simulink model "Controllo_CG"  (R2014b)
settings: Solver=ode45  SolverMode=SingleTasking  StartTime=0.0  StopTime=10.0  RelTol=1e-3
values from neighbouring files (symbols this model uses):
  b = size(G,2)    [OffsetFree.m]    (also in main.m = [qmax -qmin hmax -hmin Fmax -Fmin]')
  delta = 1e-3    (= 0.001)    [main.m]
  F_lq = F_aug(1,1:dimA(1))    [LQI_control.m]
  Fhi = sysTotal.a    [main.m]
  G = sysTotal.b    [main.m]
  Hc = [1 0 0 0 0; 0 1 0 0 0; -F_lq Ci]    [main.m]
  k0 = horizon    [calcola_k0.m]    (also in main.m = 35)
  L = [sysTotal.d; zeros(nc-1,1)]    [main.m]
  par = [1 5 1.5 4 20 0.5 1 0.5]    [main.m]
  Riferimento = [0 0 0 0 0 0 0 0 0 0 0 0 ... (1000 elements, 1x1000)]    [ref.mat]
  T = [1 0 0; -1 0 0; 0 1 0; 0 -1 0; 0 0 1; 0 0 -1]    [main.m]
  Ts = 0.01    [main.m]
  ueq = m2*g + (k2 + k1/R^2)*heq    [main.m]
  x0 = zeros(size(Ad,1),1)    [LQI_control.m]    (also in main.m = [0 0 0 0]')
  xeq = [0 0 -g*L*m1*R/k1 0]    [main.m]
undefined symbols (not defined in the file or in its folder): Ai, Bi, Calcolo_CG, Ci, Di
settings Model: CovSFcnEnable=on  Creator=Piero  LastModifiedBy=Gianni
settings OptimizationCC: BlockReduction=off  BooleanDataType=off  UseDivisionForNetSlopeComputation=off  SimCompilerOptimization=off
settings DebuggingCC: SaveWithParameterizedLinksMsg=none  UnderspecifiedInitializationDetection=Classic  MergeDetectMultiDrivingBlocksExec=none  SignalResolutionControl=TryResolveAllWithWarning  SolverPrmCheckMsg=none  FrameProcessingCompatibilityMsg=error
settings HardwareCC: TargetUnknown=on
settings RTWCC: RTWCompilerOptimization=off

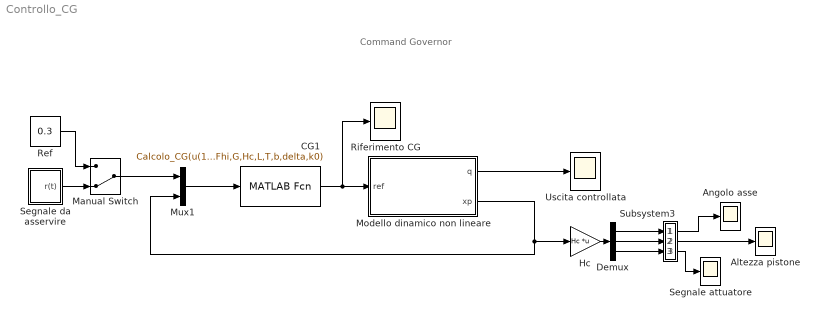
== system Controllo_CG ==
  note: Command Governor
  Altezza pistone : Scope
      settings: TimeRange=10  YMin=-1  YMax=1  SaveName=h_CG
  Angolo asse : Scope
      settings: YMin=-0.5  YMax=0.5  SaveName=q_CG
  CG1 : MATLABFcn  MATLABFcn=Calcolo_CG(u(1),u(2:6),Fhi,G,Hc,L,T,b,delta,k0)  OutputDimensions=1  SampleTime=Ts
  Demux : Demux  Outputs=3
  Hc : Gain  Gain=Hc  Multiplication=Matrix(K*u)
  Manual Switch : ManualSwitch  CurrentSetting=0
  Modello dinamico non lineare : Subsystem
  Mux1 : Mux  Inputs=2
  Ref : Constant  Value=0.3
  Riferimento CG : Scope
      settings: YMin=0.04795  YMax=0.049  SaveName=ref_CG
  Segnale attuatore : Scope
      settings: TimeRange=10  YMin=-8.353816285490428  YMax=-5.295925289307348  SaveName=u_CG
  Segnale da asservire : Subsystem
  Subsystem3 : Subsystem
      mask Display: port_label('output', 1, '')
  "Uscita controllata " : Scope
      settings: YMin=0.09  YMax=0.1325
  wires:
  Modello dinamico non lineare/2(xp) -> Mux1/2, Hc/1
  Modello dinamico non lineare/1(q) -> "Uscita controllata "/1
  Hc/1 -> Demux/1
  Manual Switch/1 -> Mux1/1
  Demux/1 -> Subsystem3/1(z)
  Demux/2 -> Subsystem3/2(h)
  Demux/3 -> Subsystem3/3(F)
  Subsystem3/1(z_vinc) -> Angolo asse/1
  Subsystem3/2(h_vinc) -> Altezza pistone/1
  Subsystem3/3(F_vinc) -> Segnale attuatore/1
  Segnale da asservire/1(r(t)) -> Manual Switch/2
  Ref/1 -> Manual Switch/1
  Mux1/1 -> CG1/1
  CG1/1 -> Riferimento CG/1, Modello dinamico non lineare/1(ref)

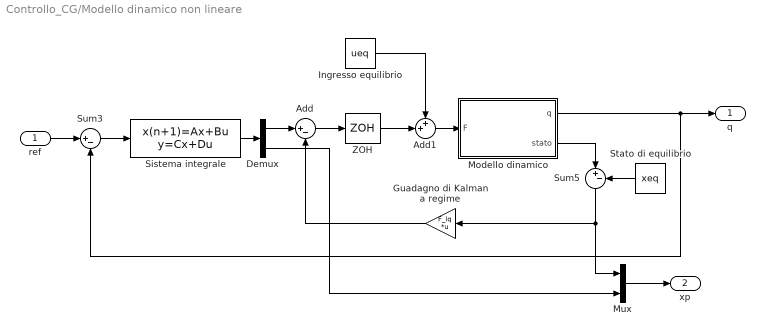
== system Controllo_CG/Modello dinamico non lineare ==
  ref : Inport
  Add : Sum  Inputs=|+-
  Add1 : Sum  Inputs=++|
  Demux : Demux  Outputs=2
  Guadagno di Kalman a regime : Gain  Gain=F_lq  Multiplication=Matrix(K*u) (u vector)
  Ingresso equilibrio : Constant  Value=ueq
  Modello dinamico : Subsystem
  Mux : Mux  Inputs=2
  Sistema integrale : DiscreteStateSpace  A=Ai  B=Bi  C=[Ci;1]  D=[Di;0]  SampleTime=Ts
  Stato di equilibrio : Constant  Value=xeq
  Sum3 : Sum  Inputs=|+-
  Sum5 : Sum  Inputs=|+-
  ZOH : ZeroOrderHold  SampleTime=Ts
  q : Outport
  xp : Outport  Port=2
  wires:
  Demux/2 -> Mux/2
  Sistema integrale/1 -> Demux/1
  Mux/1 -> xp/1
  Sum3/1 -> Sistema integrale/1
  Stato di equilibrio/1 -> Sum5/2
  ZOH/1 -> Add1/2
  Modello dinamico/1(q) -> Sum3/2, q/1
  Add/1 -> ZOH/1
  Modello dinamico/2(stato) -> Sum5/1
  ref/1 -> Sum3/1
  Add1/1 -> Modello dinamico/1("F ")
  Demux/1 -> Add/1
  Guadagno di Kalman a regime/1 -> Add/2
  Ingresso equilibrio/1 -> Add1/1
  Sum5/1 -> Mux/1, Guadagno di Kalman a regime/1

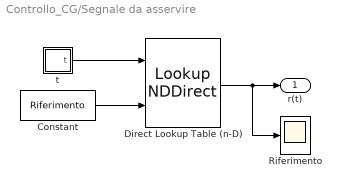
== system Controllo_CG/Segnale da asservire ==
  Constant : Constant  Value=Riferimento
  Direct Lookup Table (n-D) : LookupNDDirect  NumberOfTableDimensions=1  TableIsInput=on
  Riferimento : Scope
      settings: YMin=0.3995  YMax=0.3998  SaveName=ref
  t : Subsystem
  r(t) : Outport
  wires:
  Constant/1 -> Direct Lookup Table (n-D)/2
  t/1(t) -> Direct Lookup Table (n-D)/1
  Direct Lookup Table (n-D)/1 -> Riferimento/1, r(t)/1

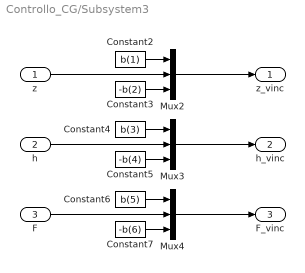
== system Controllo_CG/Subsystem3 ==
  z : Inport
  h : Inport  Port=2
  F : Inport  Port=3
  Constant2 : Constant  Value=b(1)
  Constant3 : Constant  Value=-b(2)
  Constant4 : Constant  Value=b(3)
  Constant5 : Constant  Value=-b(4)
  Constant6 : Constant  Value=b(5)
  Constant7 : Constant  Value=-b(6)
  Mux2 : Mux  Inputs=3
  Mux3 : Mux  Inputs=3
  Mux4 : Mux  Inputs=3
  z_vinc : Outport
  h_vinc : Outport  Port=2
  F_vinc : Outport  Port=3
  wires:
  h/1 -> Mux3/2
  Mux2/1 -> z_vinc/1
  F/1 -> Mux4/2
  Constant3/1 -> Mux2/3
  Constant2/1 -> Mux2/1
  z/1 -> Mux2/2
  Constant4/1 -> Mux3/1
  Constant5/1 -> Mux3/3
  Constant6/1 -> Mux4/1
  Constant7/1 -> Mux4/3
  Mux3/1 -> h_vinc/1
  Mux4/1 -> F_vinc/1

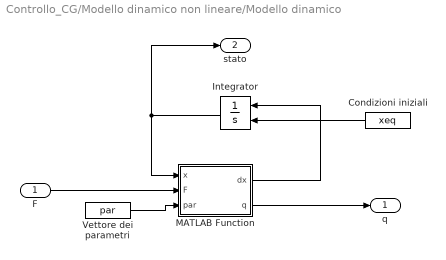
== system Controllo_CG/Modello dinamico non lineare/Modello dinamico ==
  "F " : Inport
  Condizioni iniziali : Constant  Value=xeq
  Integrator : Integrator  InitialConditionSource=external  InitialCondition=x0
  MATLAB Function : MATLAB Function  TreatAsAtomicUnit=on
  Vettore dei parametri : Constant  Value=par
  q : Outport
  stato : Outport  Port=2
  wires:
  MATLAB Function/2(q) -> q/1
  Condizioni iniziali/1 -> Integrator/2
  Vettore dei parametri/1 -> MATLAB Function/3(par)
  Integrator/1 -> MATLAB Function/1(x), stato/1
  "F "/1 -> MATLAB Function/2(F)
  MATLAB Function/1(dx) -> Integrator/1

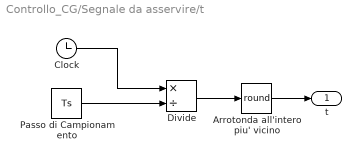
== system Controllo_CG/Segnale da asservire/t ==
  Arrotonda all'intero piu' vicino : Rounding  Operator=round
  Clock : Clock
  Divide : Product  Inputs=*/
  Passo di Campionamento : Constant  Value=Ts
  t : Outport
  wires:
  Arrotonda all'intero piu' vicino/1 -> t/1
  Divide/1 -> Arrotonda all'intero piu' vicino/1
  Passo di Campionamento/1 -> Divide/2
  Clock/1 -> Divide/1

== matlab function Controllo_CG/Modello dinamico non lineare/Modello dinamico/MATLAB Function ==
  data: x input; dx output; F input; par input; q output
function [dx, q] = sys( x, F, par )

% Assegnazione paramentri
m1 = par(1);
k1 = par(2);
b1 = par(3);
m2 = par(4);
k2 = par(5);
b2 = par(6);
L = par(7);
R = par(8);

g = 9.81;


dx = [x(2); ...
     -b1/(m1*L^2)*x(2) - k1/(m1*L^2)*(x(3)/R + x(1)) - g*cos(x(1))/L; ...
      x(4); ... 
     -b2/m2*x(4) - k2/m2*x(3) - k1/(m2*R)*(x(3)/R + x(1)) - g + F/m2];

q = x(1);

end
